simulink model "Simulink_Texto"  (R2020b)
settings: Solver=VariableStepAuto  StartTime=0.0  StopTime=Inf  RelTol=1e-3
libraries: commutil2 x2, commdigbbndpm3 x2, commchan3 x1
settings Model: Creator=enrique  LastModifiedBy=enrique
settings SFSimCC: CustomCodeUndefinedFunction=UseInterfaceOnly

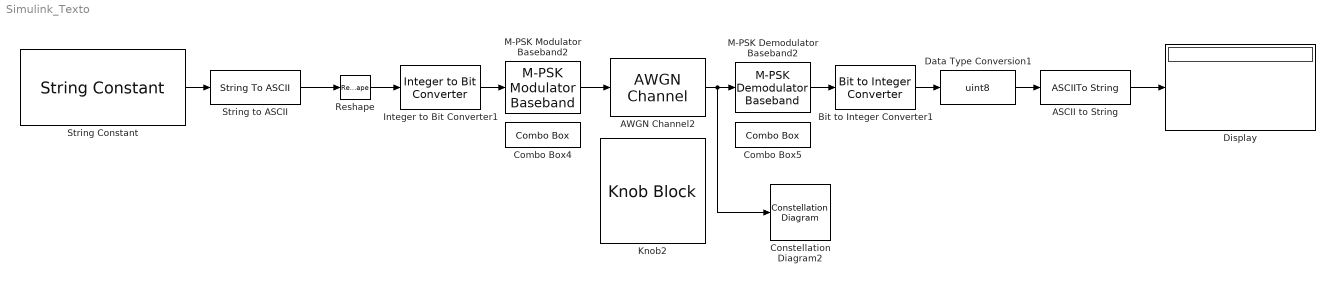
== system Simulink_Texto ==
  ASCII to String : ASCIIToString
  AWGN Channel2 : commchan3/AWGN Channel  InputProcessing=Columns as channels (frame based)  seed=67  noiseMode="Signal to noise ratio  (SNR)"  EbNodB=67  EsNodB=10  SNRdB=7.811298362604781  bitsPerSym=1  Ps=1  Tsym=1  variance=1
  Bit to Integer Converter1 : commutil2/Bit to Integer Converter  nbits=8  bitOrder=MSB first  signedOutputValues=Unsigned  outDtype=Inherit via internal rule  outDtypeSigned=Inherit via internal rule
  Combo Box4 : ComboBox  LabelPosition=Hide  SelectedLabel=M=2
      settings: Values={{'M=2', 'M=4', 'M=8', 'M=16'}, [2 4 8 16]}
  Combo Box5 : ComboBox  LabelPosition=Hide  SelectedLabel=M=2
      settings: Values={{'M=2', 'M=4', 'M=8', 'M=16'}, [2 4 8 16]}
  Constellation Diagram2 : ConstellationDiagram
  Data Type Conversion1 : DataTypeConversion  OutDataTypeStr=uint8
  Display : Display
  Integer to Bit Converter1 : commutil2/Integer to Bit Converter  nbits=8  signedInputValues=Unsigned  bitOrder=MSB first  outDtype=Inherit via internal rule
  Knob2 : KnobBlock  ScaleMin=-50  ScaleMax=50
  M-PSK Demodulator Baseband2 : commdigbbndpm3/M-PSK Demodulator Baseband  M=2  OutType=Bit  DecType=Hard decision  VarSource=Dialog  Variance=1  Dec=Gray  Mapping=[0:7]  Ph=0  outDtype1=Inherit via internal rule  outDtype2=Inherit via internal rule  derotateFactorWordLen=16  derotateFactorDataTypeStr=Inherit: Same word length as input  derotateFactorLastDataTypeStr=Inherit: Same word length as input
  M-PSK Modulator Baseband2 : commdigbbndpm3/M-PSK Modulator Baseband  M=2  InType=Bit  Enc=Gray  Mapping=[0:7]  Ph=0  outDtype=double  outWordLen=16  outUDDataType=sfix(16)  outFracLenMode=Best precision  outFracLen=15  outDataTypeStr=double  outLastDataTypeStr=double
  Reshape : Reshape
  String Constant : StringConstant  String="\"¿Hay vida más allá de TC?\""
  String to ASCII : StringToASCII  OutputVectorSize=16*3
  wires:
  M-PSK Demodulator Baseband2/1 -> Bit to Integer Converter1/1
  Integer to Bit Converter1/1 -> M-PSK Modulator Baseband2/1
  M-PSK Modulator Baseband2/1 -> AWGN Channel2/1
  AWGN Channel2/1 -> M-PSK Demodulator Baseband2/1, Constellation Diagram2/1
  Bit to Integer Converter1/1 -> Data Type Conversion1/1
  Data Type Conversion1/1 -> ASCII to String/1
  Reshape/1 -> Integer to Bit Converter1/1
  ASCII to String/1 -> Display/1
  String to ASCII/1 -> Reshape/1
  String Constant/1 -> String to ASCII/1
